simulink model "nonLin_Model_std_V2"  (R2023b)
settings: Solver=ode23t  StartTime=0.0  StopTime=Tend  FixedStep=Ts  MaxStep=0.002  RelTol=1e-3
InitFcn:
  | sysParam = load("sysParam.mat");
  | load('./zz_temp/controlletTypeToUse.mat')
undefined symbols (not defined in the file): C, sysID
libraries: slpidlib x12, cstblocks x2
(part 1 of 2)
settings Model: Creator=maxja  LastModifiedBy=maxja

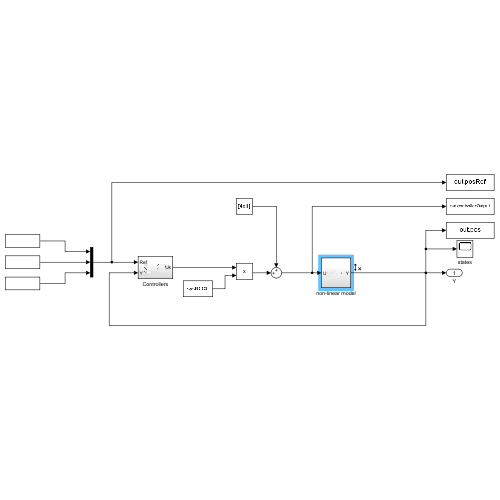
[thumbnail: Simulink's stored preview of the top-level diagram]
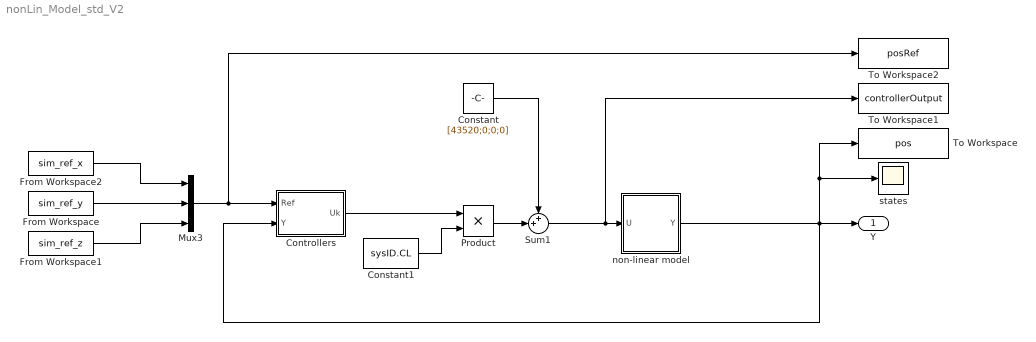
== system nonLin_Model_std_V2 ==
  Constant : Constant  Value=[43520;0;0;0]
  Constant1 : Constant  Value=sysID.CL
  Controllers : Subsystem
  From Workspace : FromWorkspace  VariableName=sim_ref_y
  From Workspace1 : FromWorkspace  VariableName=sim_ref_z
  From Workspace2 : FromWorkspace  VariableName=sim_ref_x
  Mux3 : Mux  Inputs=3
  Product : Product
  Sum1 : Sum  Inputs=++|
  To Workspace : ToWorkspace  VariableName=pos  SaveFormat=Timeseries  SampleTime=-1
  To Workspace1 : ToWorkspace  VariableName=controllerOutput  SaveFormat=Timeseries  SampleTime=-1
  To Workspace2 : ToWorkspace  VariableName=posRef  SaveFormat=Timeseries  SampleTime=-1
  non-linear model : Subsystem
  states : Scope
  Y : Outport
  wires:
  non-linear model/1(Y) -> To Workspace/1, states/1, Controllers/2(Y), Y/1
  From Workspace2/1 -> Mux3/1
  From Workspace/1 -> Mux3/2
  From Workspace1/1 -> Mux3/3
  Sum1/1 -> To Workspace1/1, non-linear model/1(U)
  Mux3/1 -> To Workspace2/1, Controllers/1(Ref)
  Controllers/1(Uk) -> Product/1
  Constant/1 -> Sum1/1
  Product/1 -> Sum1/2
  Constant1/1 -> Product/2

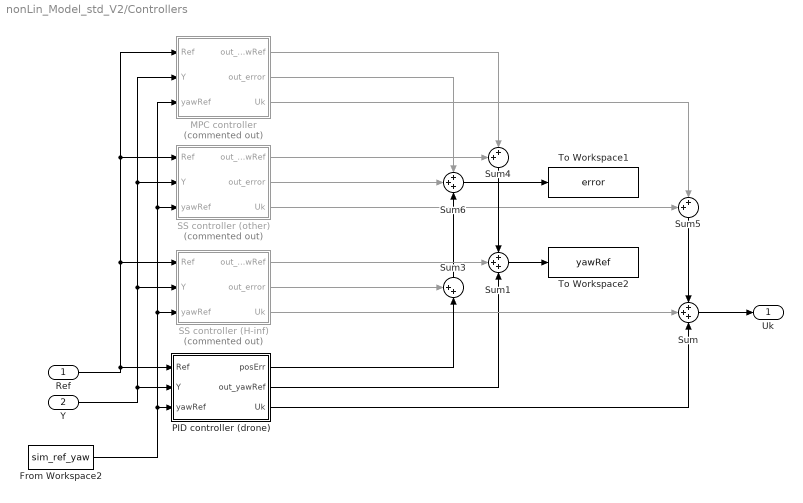
== system nonLin_Model_std_V2/Controllers ==
  Ref : Inport
  Y : Inport  Port=2
  From Workspace2 : FromWorkspace  VariableName=sim_ref_yaw
  MPC controller : Subsystem  Commented=on
  PID controller (drone) : Subsystem
  SS controller (H-inf) : Subsystem  Commented=on
  SS controller (other) : Subsystem  Commented=on
  Sum : Sum  Inputs=+++
  Sum1 : Sum  Inputs=+++
  Sum3 : Sum  Inputs=++|
  Sum4 : Sum  Inputs=++|
  Sum5 : Sum  Inputs=++|
  Sum6 : Sum  Inputs=+++
  To Workspace1 : ToWorkspace  VariableName=error  SaveFormat=Timeseries  SampleTime=-1
  To Workspace2 : ToWorkspace  VariableName=yawRef  SaveFormat=Timeseries  SampleTime=-1
  Uk : Outport
  wires:
  Y/1 -> PID controller (drone)/2(Y), SS controller (H-inf)/2(Y), MPC controller/2(Y), SS controller (other)/2(Y)
  Ref/1 -> PID controller (drone)/1(Ref), MPC controller/1(Ref), SS controller (other)/1(Ref), SS controller (H-inf)/1(Ref)
  SS controller (other)/3(Uk) -> Sum5/1
  PID controller (drone)/3(Uk) -> Sum/3
  From Workspace2/1 -> MPC controller/3(yawRef), SS controller (other)/3(yawRef), SS controller (H-inf)/3(yawRef), PID controller (drone)/3(yawRef)
  SS controller (other)/1(out_yawRef) -> Sum4/1
  SS controller (other)/2(out_error) -> Sum6/2
  Sum6/1 -> To Workspace1/1
  Sum1/1 -> To Workspace2/1
  PID controller (drone)/2(out_yawRef) -> Sum1/3
  SS controller (H-inf)/3(Uk) -> Sum/2
  Sum3/1 -> Sum6/3
  PID controller (drone)/1(posErr) -> Sum3/2
  MPC controller/1(out_yawRef) -> Sum4/2
  Sum4/1 -> Sum1/1
  Sum5/1 -> Sum/1
  MPC controller/3(Uk) -> Sum5/2
  MPC controller/2(out_error) -> Sum6/1
  SS controller (H-inf)/1(out_yawRef) -> Sum1/2
  SS controller (H-inf)/2(out_error) -> Sum3/1
  Sum/1 -> Uk/1

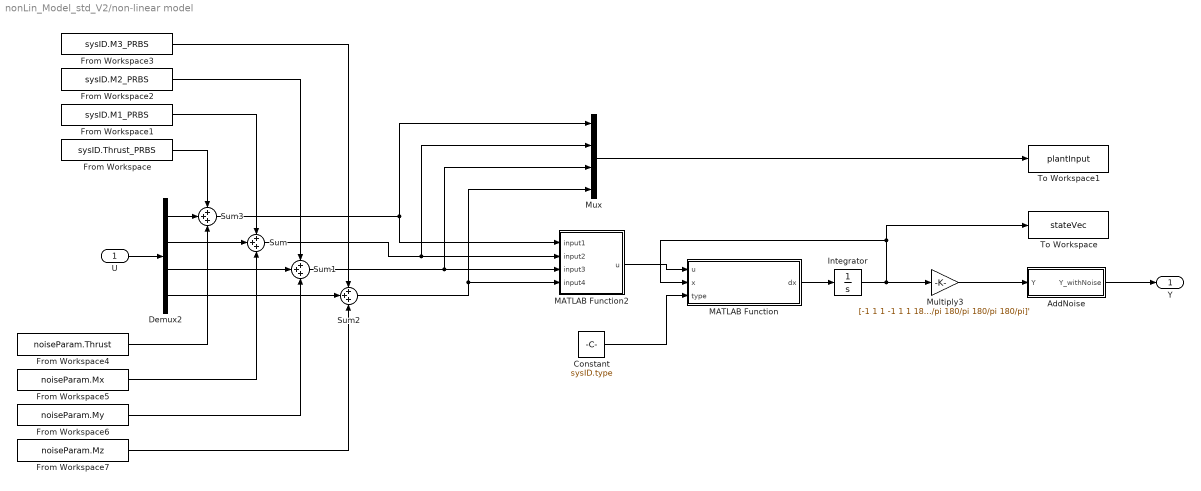
== system nonLin_Model_std_V2/non-linear model ==
  U : Inport  PortDimensions=4
  AddNoise : Subsystem
  Constant : Constant  Value=sysID.type
  Demux2 : Demux
  From Workspace : FromWorkspace  VariableName=sysID.Thrust_PRBS
  From Workspace1 : FromWorkspace  VariableName=sysID.M1_PRBS
  From Workspace2 : FromWorkspace  VariableName=sysID.M2_PRBS
  From Workspace3 : FromWorkspace  VariableName=sysID.M3_PRBS
  From Workspace4 : FromWorkspace  VariableName=noiseParam.Thrust
  From Workspace5 : FromWorkspace  VariableName=noiseParam.Mx
  From Workspace6 : FromWorkspace  VariableName=noiseParam.My
  From Workspace7 : FromWorkspace  VariableName=noiseParam.Mz
  Integrator : Integrator  InitialCondition=[0;0;0;0;0;0;0;0;0;0;0;0]  LimitOutput=on  UpperSaturationLimit=[inf inf inf inf inf inf inf inf inf inf inf inf]'  LowerSaturationLimit=-[inf inf 0 inf inf inf inf inf inf inf inf inf]'
  MATLAB Function : MATLAB Function  TreatAsAtomicUnit=on
  MATLAB Function2 : MATLAB Function  TreatAsAtomicUnit=on
  Multiply3 : Gain  Gain=[-1 1 1 -1 1 1 180/pi 180/pi 180/pi 180/pi 180/pi 180/pi]'
  Mux : Mux
  Sum{,1..3} (4 alike) : Sum  Inputs=+++
  To Workspace : ToWorkspace  VariableName=stateVec  SaveFormat=Timeseries  SampleTime=-1
  To Workspace1 : ToWorkspace  VariableName=plantInput  SaveFormat=Timeseries  SampleTime=-1
  Y : Outport
  wires:
  MATLAB Function/1(dx) -> Integrator/1
  U/1 -> Demux2/1
  Sum/1 -> Mux/2, MATLAB Function2/2(input2)
  Sum3/1 -> MATLAB Function2/1(input1), Mux/1
  Sum1/1 -> MATLAB Function2/3(input3), Mux/3
  Sum2/1 -> MATLAB Function2/4(input4), Mux/4
  From Workspace5/1 -> Sum/3
  From Workspace6/1 -> Sum1/3
  From Workspace7/1 -> Sum2/3
  From Workspace/1 -> Sum3/1
  From Workspace1/1 -> Sum/1
  From Workspace2/1 -> Sum1/1
  From Workspace3/1 -> Sum2/1
  Constant/1 -> MATLAB Function/3(type)
  Demux2/2 -> Sum/2
  Demux2/4 -> Sum2/2
  Demux2/3 -> Sum1/2
  Demux2/1 -> Sum3/2
  Multiply3/1 -> AddNoise/1(Y)
  MATLAB Function2/1(u) -> MATLAB Function/1(u)
  Mux/1 -> To Workspace1/1
  AddNoise/1(Y_withNoise) -> Y/1
  From Workspace4/1 -> Sum3/3
  Integrator/1 -> Multiply3/1, To Workspace/1, MATLAB Function/2(x)

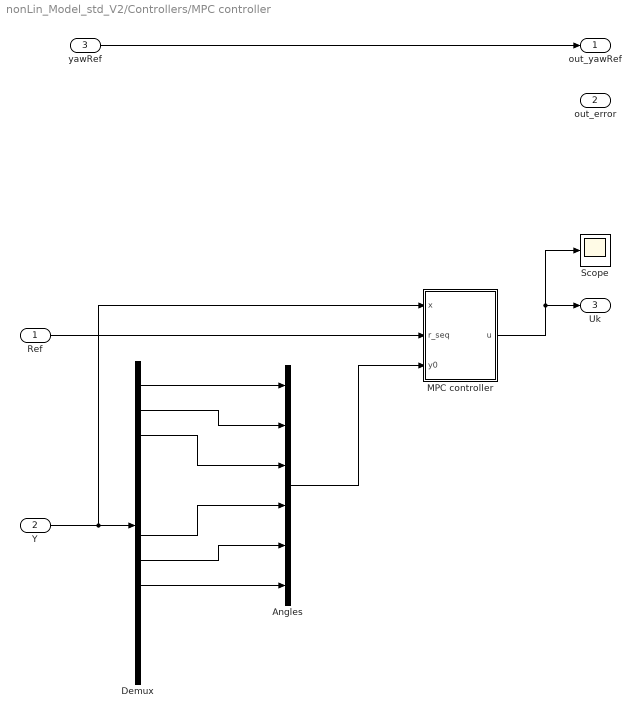
== system nonLin_Model_std_V2/Controllers/MPC controller ==
  Ref : Inport
  Y : Inport  Port=2
  yawRef : Inport  Port=3
  Angles : Mux  Inputs=6
  Demux : Demux  Outputs=12
  MPC controller : MATLAB Function  TreatAsAtomicUnit=on
  Scope : Scope
  out_yawRef : Outport
  out_error : Outport  Port=2
  Uk : Outport  Port=3
  wires:
  MPC controller/1(u) -> Scope/1, Uk/1
  Demux/7 -> Angles/4
  yawRef/1 -> out_yawRef/1
  Demux/9 -> Angles/6
  Demux/1 -> Angles/1
  Demux/3 -> Angles/3
  Demux/2 -> Angles/2
  Y/1 -> MPC controller/1(x), Demux/1
  Ref/1 -> MPC controller/2(r_seq)
  Demux/8 -> Angles/5
  Angles/1 -> MPC controller/3(y0)

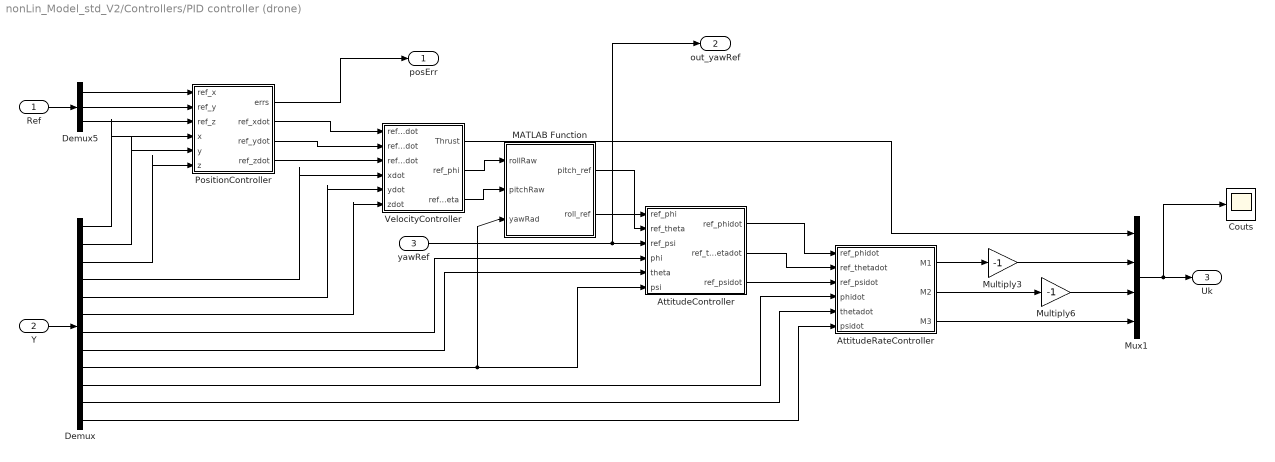
== system nonLin_Model_std_V2/Controllers/PID controller (drone) ==
  Ref : Inport
  Y : Inport  Port=2
  yawRef : Inport  Port=3
  AttitudeController : Subsystem
  AttitudeRateController : Subsystem
  Couts : Scope
  Demux : Demux  Outputs=12
  Demux5 : Demux  Outputs=3
  MATLAB Function : MATLAB Function  TreatAsAtomicUnit=on
  Multiply3 : Gain  Gain=-1
  Multiply6 : Gain  Gain=-1
  Mux1 : Mux
  PositionController : Subsystem
  VelocityController : Subsystem
  posErr : Outport
  out_yawRef : Outport  Port=2
  Uk : Outport  Port=3
  wires:
  Y/1 -> Demux/1
  Demux/1 -> PositionController/4(x)
  Demux/2 -> PositionController/5(y)
  Demux/3 -> PositionController/6(z)
  Demux/12 -> AttitudeRateController/6(psidot)
  Demux/11 -> AttitudeRateController/5(thetadot)
  Demux/10 -> AttitudeRateController/4(phidot)
  Demux/9 -> MATLAB Function/3(yawRad), AttitudeController/6(psi)
  Demux/6 -> VelocityController/6(zdot)
  Demux/5 -> VelocityController/5(ydot)
  Demux/4 -> VelocityController/4(xdot)
  Demux5/1 -> PositionController/1(ref_x)
  Demux5/2 -> PositionController/2(ref_y)
  Demux5/3 -> PositionController/3(ref_z)
  Ref/1 -> Demux5/1
  PositionController/2(ref_xdot) -> VelocityController/1(ref_xdot)
  PositionController/3(ref_ydot) -> VelocityController/2(ref_ydot)
  PositionController/4(ref_zdot) -> VelocityController/3(ref_zdot)
  yawRef/1 -> out_yawRef/1, AttitudeController/3(ref_psi)
  AttitudeController/3(ref_psidot) -> AttitudeRateController/3(ref_psidot)
  AttitudeController/2(ref_thetadot) -> AttitudeRateController/2(ref_thetadot)
  AttitudeController/1(ref_phidot) -> AttitudeRateController/1(ref_phidot)
  AttitudeRateController/1(M1) -> Multiply3/1
  AttitudeRateController/3(M3) -> Mux1/4
  VelocityController/1(Thrust) -> Mux1/1
  Mux1/1 -> Couts/1, Uk/1
  Multiply3/1 -> Mux1/2
  AttitudeRateController/2(M2) -> Multiply6/1
  Multiply6/1 -> Mux1/3
  Demux/7 -> AttitudeController/4(phi)
  Demux/8 -> AttitudeController/5(theta)
  VelocityController/2(ref_phi) -> MATLAB Function/1(rollRaw)
  VelocityController/3(ref_theta) -> MATLAB Function/2(pitchRaw)
  MATLAB Function/1(pitch_ref) -> AttitudeController/2(ref_theta)
  MATLAB Function/2(roll_ref) -> AttitudeController/1(ref_phi)
  PositionController/1(errs) -> posErr/1

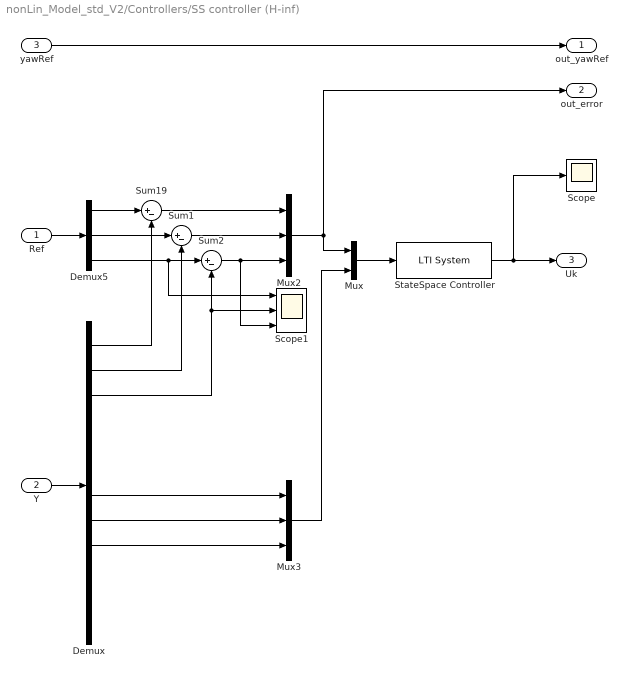
== system nonLin_Model_std_V2/Controllers/SS controller (H-inf) ==
  Ref : Inport
  Y : Inport  Port=2
  yawRef : Inport  Port=3
  Demux : Demux  Outputs=12
  Demux5 : Demux  Outputs=3
  Mux : Mux  Inputs=2
  Mux2 : Mux  Inputs=3
  Mux3 : Mux  Inputs=3
  Scope : Scope
  Scope1 : Scope  NumInputPorts=3
  StateSpace Controller : cstblocks/LTI System  sys=K  IC=[]  PadeOrder=0
  Sum1 : Sum  Inputs=|+-
  Sum19 : Sum  Inputs=|+-
  Sum2 : Sum  Inputs=|+-
  out_yawRef : Outport
  out_error : Outport  Port=2
  Uk : Outport  Port=3
  wires:
  Y/1 -> Demux/1
  Ref/1 -> Demux5/1
  Demux5/1 -> Sum19/1
  Demux5/2 -> Sum1/1
  Demux/3 -> Sum2/2, Scope1/2
  Demux/2 -> Sum1/2
  Sum19/1 -> Mux2/1
  Demux/1 -> Sum19/2
  Demux5/3 -> Scope1/1, Sum2/1
  Sum1/1 -> Mux2/2
  Sum2/1 -> Scope1/3, Mux2/3
  yawRef/1 -> out_yawRef/1
  Demux/9 -> Mux3/3
  Mux2/1 -> out_error/1, Mux/1
  Demux/7 -> Mux3/1
  Demux/8 -> Mux3/2
  Mux3/1 -> Mux/2
  Mux/1 -> StateSpace Controller/1
  StateSpace Controller/1 -> Uk/1, Scope/1

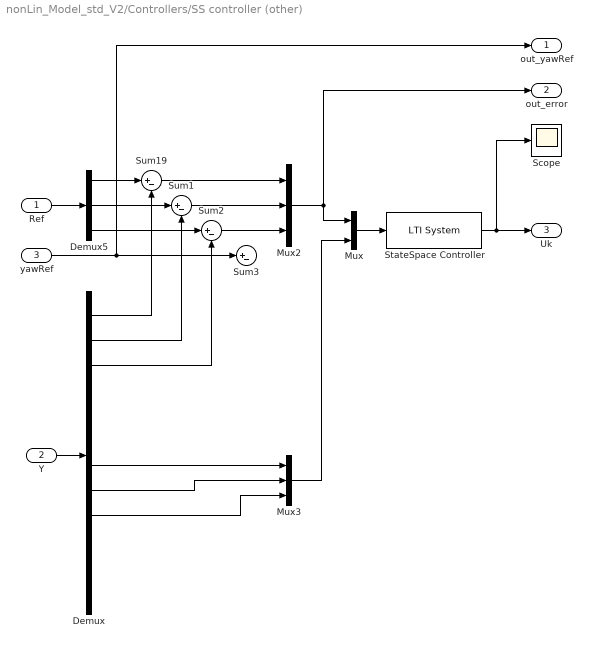
== system nonLin_Model_std_V2/Controllers/SS controller (other) ==
  Ref : Inport
  Y : Inport  Port=2
  yawRef : Inport  Port=3
  Demux : Demux  Outputs=12
  Demux5 : Demux  Outputs=3
  Mux : Mux  Inputs=2
  Mux2 : Mux  Inputs=3
  Mux3 : Mux  Inputs=3
  Scope : Scope
  StateSpace Controller : cstblocks/LTI System  sys=K  IC=[]  PadeOrder=0
  Sum{1..3,19} (4 alike) : Sum  Inputs=|+-
  out_yawRef : Outport
  out_error : Outport  Port=2
  Uk : Outport  Port=3
  wires:
  Y/1 -> Demux/1
  Ref/1 -> Demux5/1
  Demux5/1 -> Sum19/1
  Demux5/2 -> Sum1/1
  Demux/3 -> Sum2/2
  Demux/2 -> Sum1/2
  Sum19/1 -> Mux2/1
  Demux/1 -> Sum19/2
  Demux5/3 -> Sum2/1
  Sum1/1 -> Mux2/2
  Sum2/1 -> Mux2/3
  yawRef/1 -> out_yawRef/1, Sum3/1
  Demux/9 -> Mux3/3
  Mux2/1 -> Mux/1, out_error/1
  Demux/7 -> Mux3/1
  Demux/8 -> Mux3/2
  Mux3/1 -> Mux/2
  Mux/1 -> StateSpace Controller/1
  StateSpace Controller/1 -> Scope/1, Uk/1

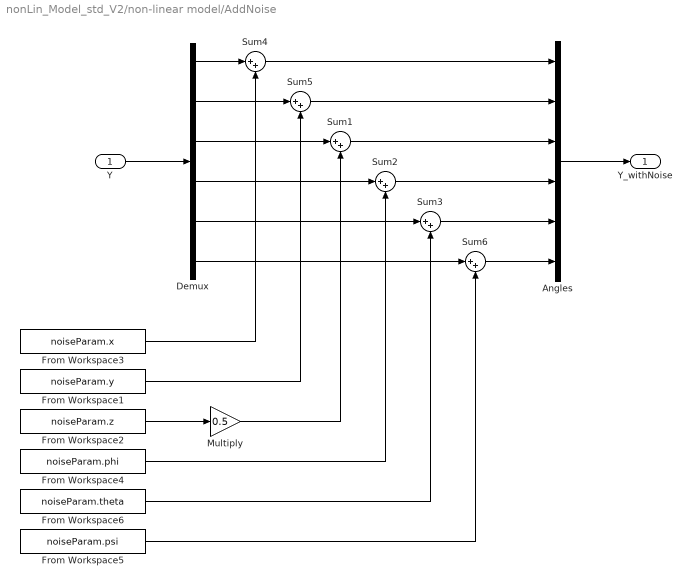
== system nonLin_Model_std_V2/non-linear model/AddNoise ==
  Y : Inport
  Angles : Mux  Inputs=6
  Demux : Demux  Outputs=6
  From Workspace1 : FromWorkspace  VariableName=noiseParam.y
  From Workspace2 : FromWorkspace  VariableName=noiseParam.z
  From Workspace3 : FromWorkspace  VariableName=noiseParam.x
  From Workspace4 : FromWorkspace  VariableName=noiseParam.phi
  From Workspace5 : FromWorkspace  VariableName=noiseParam.psi
  From Workspace6 : FromWorkspace  VariableName=noiseParam.theta
  Multiply : Gain  Gain=0.5
  Sum{1..6} (6 alike) : Sum  Inputs=|++
  Y_withNoise : Outport
  wires:
  Demux/2 -> Sum5/1
  Demux/6 -> Sum6/1
  Demux/1 -> Sum4/1
  Demux/3 -> Sum1/1
  Demux/4 -> Sum2/1
  Demux/5 -> Sum3/1
  Sum4/1 -> Angles/1
  Sum6/1 -> Angles/6
  Sum3/1 -> Angles/5
  Sum2/1 -> Angles/4
  Sum1/1 -> Angles/3
  Sum5/1 -> Angles/2
  Y/1 -> Demux/1
  Angles/1 -> Y_withNoise/1
  From Workspace3/1 -> Sum4/2
  From Workspace1/1 -> Sum5/2
  From Workspace2/1 -> Multiply/1
  From Workspace4/1 -> Sum2/2
  From Workspace6/1 -> Sum3/2
  From Workspace5/1 -> Sum6/2
  Multiply/1 -> Sum1/2

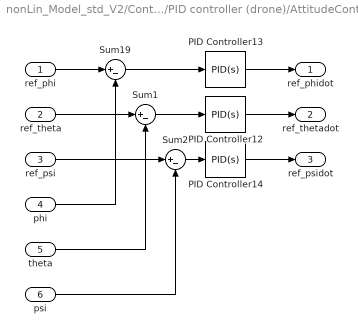
== system nonLin_Model_std_V2/Controllers/PID controller (drone)/AttitudeController ==
  ref_phi : Inport
  ref_theta : Inport  Port=2
  ref_psi : Inport  Port=3
  phi : Inport  Port=4
  theta : Inport  Port=5
  psi : Inport  Port=6
  PID Controller12 : slpidlib/PID Controller  Controller=PID  Form=Parallel  TimeDomain=Continuous-time  UseExternalTs=off  SampleTime=-1  IntegratorMethod=Forward Euler  FilterMethod=Forward Euler  ControllerParametersSource=internal  P=C.att.theta.Kp  I=C.att.theta.Ki  UseKiTs=off  D=C.att.theta.Kd  N=100  UseFilter=on  TunerSelectOption=Transfer Function Based (PID Tuner App)  InitialConditionSource=internal  InitialConditionForIntegrator=0  InitialConditionForFilter=0  DifferentiatorICPrevScaledInput=0  ExternalReset=none  TrackingMode=off  Kt=1  LimitOutput=off  SatLimitsSource=internal  UpperSaturationLimit=inf  LowerSaturationLimit=-inf  LinearizeAsGain=on  AntiWindupMode=none  Kb=1  LimitIntegrator=off  UpperIntegratorSaturationLimit=inf  LowerIntegratorSaturationLimit=-inf  POutMin=[]  POutMax=[]  IOutMin=[]  IOutMax=[]  DOutMin=[]  DOutMax=[]  NOutMin=[]  NOutMax=[]  SumOutMin=[]  SumOutMax=[]  SaturationOutMin=[]  SaturationOutMax=[]  PParamMin=[]  PParamMax=[]  IParamMin=[]  IParamMax=[]  DParamMin=[]  DParamMax=[]  NParamMin=[]  NParamMax=[]  KbParamMin=[]  KbParamMax=[]  KtParamMin=[]  KtParamMax=[]  KbOutMin=[]  KbOutMax=[]  KtOutMin=[]  KtOutMax=[]  IntegratorOutMin=[]  IntegratorOutMax=[]  FilterOutMin=[]  FilterOutMax=[]  SumI1OutMin=[]  SumI1OutMax=[]  SumI2OutMin=[]  SumI2OutMax=[]  SumI3OutMin=[]  SumI3OutMax=[]  SumI4OutMin=[]  SumI4OutMax=[]  SumDOutMin=[]  SumDOutMax=[]  DifferentiatorOutMin=[]  DifferentiatorOutMax=[]  FilterDiffOutCoefMin=[]  FilterDiffOutCoefMax=[]  ReciprocalOutMin=[]  ReciprocalOutMax=[]  SumDenOutMin=[]  SumDenOutMax=[]  SumNumOutMin=[]  SumNumOutMax=[]  DivideOutMin=[]  DivideOutMax=[]  UdiffTsProdOutMin=[]  UdiffTsProdOutMax=[]  NTsProdOutMin=[]  NTsProdOutMax=[]  UintegralTsProdOutMin=[]  UintegralTsProdOutMax=[]  UngainTsProdOutMin=[]  UngainTsProdOutMax=[]  ClampingZeroOutDataTypeStr=Inherit: Inherit via back propagation  ClampingZeroOutMin=[]  ClampingZeroOutMax=[]  FilterDenConstantOutDataTypeStr=Inherit: Inherit via back propagation  FilterDenConstantOutMin=[]  FilterDenConstantOutMax=[]  PCopyOutDataTypeStr=Inherit: Inherit via back propagation  PCopyOutMin=[]  PCopyOutMax=[]  NCopyOutDataTypeStr=Inherit: Inherit via back propagation  NCopyOutMin=[]  NCopyOutMax=[]  IntegratorContinuousStateAttributes=''  IntegratorStateMustResolveToSignalObject=off  IntegratorRTWStateStorageClass=Auto  FilterContinuousStateAttributes=''  FilterStateMustResolveToSignalObject=off  FilterRTWStateStorageClass=Auto  ParallelPVariant=InternalParameters  IdealPVariant=Disabled  IVariant=InternalParameters  DVariant=InternalParameters  IntegratorVariant=Continuous  SatVariant=Disabled  AWVariant=Passthrough  PCopyVariant=Disabled  TRVariant=Disabled  FdbkBlocksVariant=Forward  IdealPFdbkVariant=Disabled  SatFdbkVariant=Disabled  DerivativeFilterVariant=ContFilter  NVariant=InternalParameters  NCopyVariant=Disabled  FilterICVariant=InternalICsFilter  IntegratorICVariant=InternalICs  ExternalResetVariant=Disabled  TRSumVariant=Passthrough  SumFdbkVariant=Disabled  SumVariant=Sum_PID  TsampFilterVariant=InternalTs  TsampNgainVariant=Passthrough  TsampIntegralVariant=Disabled_SignalSpec  ExternalSaturationOutDataTypeStr=Inherit: Same as second input
  PID Controller13 : slpidlib/PID Controller  Controller=PID  Form=Parallel  TimeDomain=Continuous-time  UseExternalTs=off  SampleTime=-1  IntegratorMethod=Forward Euler  FilterMethod=Forward Euler  ControllerParametersSource=internal  P=C.att.phi.Kp  I=C.att.phi.Ki  UseKiTs=off  D=C.att.phi.Kd  N=100  UseFilter=on  TunerSelectOption=Transfer Function Based (PID Tuner App)  InitialConditionSource=internal  InitialConditionForIntegrator=0  InitialConditionForFilter=0  DifferentiatorICPrevScaledInput=0  ExternalReset=none  TrackingMode=off  Kt=1  LimitOutput=off  SatLimitsSource=internal  UpperSaturationLimit=inf  LowerSaturationLimit=-inf  LinearizeAsGain=on  AntiWindupMode=none  Kb=1  LimitIntegrator=off  UpperIntegratorSaturationLimit=inf  LowerIntegratorSaturationLimit=-inf  POutMin=[]  POutMax=[]  IOutMin=[]  IOutMax=[]  DOutMin=[]  DOutMax=[]  NOutMin=[]  NOutMax=[]  SumOutMin=[]  SumOutMax=[]  SaturationOutMin=[]  SaturationOutMax=[]  PParamMin=[]  PParamMax=[]  IParamMin=[]  IParamMax=[]  DParamMin=[]  DParamMax=[]  NParamMin=[]  NParamMax=[]  KbParamMin=[]  KbParamMax=[]  KtParamMin=[]  KtParamMax=[]  KbOutMin=[]  KbOutMax=[]  KtOutMin=[]  KtOutMax=[]  IntegratorOutMin=[]  IntegratorOutMax=[]  FilterOutMin=[]  FilterOutMax=[]  SumI1OutMin=[]  SumI1OutMax=[]  SumI2OutMin=[]  SumI2OutMax=[]  SumI3OutMin=[]  SumI3OutMax=[]  SumI4OutMin=[]  SumI4OutMax=[]  SumDOutMin=[]  SumDOutMax=[]  DifferentiatorOutMin=[]  DifferentiatorOutMax=[]  FilterDiffOutCoefMin=[]  FilterDiffOutCoefMax=[]  ReciprocalOutMin=[]  ReciprocalOutMax=[]  SumDenOutMin=[]  SumDenOutMax=[]  SumNumOutMin=[]  SumNumOutMax=[]  DivideOutMin=[]  DivideOutMax=[]  UdiffTsProdOutMin=[]  UdiffTsProdOutMax=[]  NTsProdOutMin=[]  NTsProdOutMax=[]  UintegralTsProdOutMin=[]  UintegralTsProdOutMax=[]  UngainTsProdOutMin=[]  UngainTsProdOutMax=[]  ClampingZeroOutDataTypeStr=Inherit: Inherit via back propagation  ClampingZeroOutMin=[]  ClampingZeroOutMax=[]  FilterDenConstantOutDataTypeStr=Inherit: Inherit via back propagation  FilterDenConstantOutMin=[]  FilterDenConstantOutMax=[]  PCopyOutDataTypeStr=Inherit: Inherit via back propagation  PCopyOutMin=[]  PCopyOutMax=[]  NCopyOutDataTypeStr=Inherit: Inherit via back propagation  NCopyOutMin=[]  NCopyOutMax=[]  IntegratorContinuousStateAttributes=''  IntegratorStateMustResolveToSignalObject=off  IntegratorRTWStateStorageClass=Auto  FilterContinuousStateAttributes=''  FilterStateMustResolveToSignalObject=off  FilterRTWStateStorageClass=Auto  ParallelPVariant=InternalParameters  IdealPVariant=Disabled  IVariant=InternalParameters  DVariant=InternalParameters  IntegratorVariant=Continuous  SatVariant=Disabled  AWVariant=Passthrough  PCopyVariant=Disabled  TRVariant=Disabled  FdbkBlocksVariant=Forward  IdealPFdbkVariant=Disabled  SatFdbkVariant=Disabled  DerivativeFilterVariant=ContFilter  NVariant=InternalParameters  NCopyVariant=Disabled  FilterICVariant=InternalICsFilter  IntegratorICVariant=InternalICs  ExternalResetVariant=Disabled  TRSumVariant=Passthrough  SumFdbkVariant=Disabled  SumVariant=Sum_PID  TsampFilterVariant=InternalTs  TsampNgainVariant=Passthrough  TsampIntegralVariant=Disabled_SignalSpec  ExternalSaturationOutDataTypeStr=Inherit: Same as second input
  PID Controller14 : slpidlib/PID Controller  Controller=PID  Form=Parallel  TimeDomain=Continuous-time  UseExternalTs=off  SampleTime=-1  IntegratorMethod=Forward Euler  FilterMethod=Forward Euler  ControllerParametersSource=internal  P=C.att.psi.Kp  I=C.att.psi.Ki  UseKiTs=off  D=C.att.psi.Kd  N=100  UseFilter=on  TunerSelectOption=Transfer Function Based (PID Tuner App)  InitialConditionSource=internal  InitialConditionForIntegrator=0  InitialConditionForFilter=0  DifferentiatorICPrevScaledInput=0  ExternalReset=none  TrackingMode=off  Kt=1  LimitOutput=off  SatLimitsSource=internal  UpperSaturationLimit=inf  LowerSaturationLimit=-inf  LinearizeAsGain=on  AntiWindupMode=none  Kb=1  LimitIntegrator=off  UpperIntegratorSaturationLimit=inf  LowerIntegratorSaturationLimit=-inf  POutMin=[]  POutMax=[]  IOutMin=[]  IOutMax=[]  DOutMin=[]  DOutMax=[]  NOutMin=[]  NOutMax=[]  SumOutMin=[]  SumOutMax=[]  SaturationOutMin=[]  SaturationOutMax=[]  PParamMin=[]  PParamMax=[]  IParamMin=[]  IParamMax=[]  DParamMin=[]  DParamMax=[]  NParamMin=[]  NParamMax=[]  KbParamMin=[]  KbParamMax=[]  KtParamMin=[]  KtParamMax=[]  KbOutMin=[]  KbOutMax=[]  KtOutMin=[]  KtOutMax=[]  IntegratorOutMin=[]  IntegratorOutMax=[]  FilterOutMin=[]  FilterOutMax=[]  SumI1OutMin=[]  SumI1OutMax=[]  SumI2OutMin=[]  SumI2OutMax=[]  SumI3OutMin=[]  SumI3OutMax=[]  SumI4OutMin=[]  SumI4OutMax=[]  SumDOutMin=[]  SumDOutMax=[]  DifferentiatorOutMin=[]  DifferentiatorOutMax=[]  FilterDiffOutCoefMin=[]  FilterDiffOutCoefMax=[]  ReciprocalOutMin=[]  ReciprocalOutMax=[]  SumDenOutMin=[]  SumDenOutMax=[]  SumNumOutMin=[]  SumNumOutMax=[]  DivideOutMin=[]  DivideOutMax=[]  UdiffTsProdOutMin=[]  UdiffTsProdOutMax=[]  NTsProdOutMin=[]  NTsProdOutMax=[]  UintegralTsProdOutMin=[]  UintegralTsProdOutMax=[]  UngainTsProdOutMin=[]  UngainTsProdOutMax=[]  ClampingZeroOutDataTypeStr=Inherit: Inherit via back propagation  ClampingZeroOutMin=[]  ClampingZeroOutMax=[]  FilterDenConstantOutDataTypeStr=Inherit: Inherit via back propagation  FilterDenConstantOutMin=[]  FilterDenConstantOutMax=[]  PCopyOutDataTypeStr=Inherit: Inherit via back propagation  PCopyOutMin=[]  PCopyOutMax=[]  NCopyOutDataTypeStr=Inherit: Inherit via back propagation  NCopyOutMin=[]  NCopyOutMax=[]  IntegratorContinuousStateAttributes=''  IntegratorStateMustResolveToSignalObject=off  IntegratorRTWStateStorageClass=Auto  FilterContinuousStateAttributes=''  FilterStateMustResolveToSignalObject=off  FilterRTWStateStorageClass=Auto  ParallelPVariant=InternalParameters  IdealPVariant=Disabled  IVariant=InternalParameters  DVariant=InternalParameters  IntegratorVariant=Continuous  SatVariant=Disabled  AWVariant=Passthrough  PCopyVariant=Disabled  TRVariant=Disabled  FdbkBlocksVariant=Forward  IdealPFdbkVariant=Disabled  SatFdbkVariant=Disabled  DerivativeFilterVariant=ContFilter  NVariant=InternalParameters  NCopyVariant=Disabled  FilterICVariant=InternalICsFilter  IntegratorICVariant=InternalICs  ExternalResetVariant=Disabled  TRSumVariant=Passthrough  SumFdbkVariant=Disabled  SumVariant=Sum_PID  TsampFilterVariant=InternalTs  TsampNgainVariant=Passthrough  TsampIntegralVariant=Disabled_SignalSpec  ExternalSaturationOutDataTypeStr=Inherit: Same as second input
  Sum1 : Sum  Inputs=|+-
  Sum19 : Sum  Inputs=|+-
  Sum2 : Sum  Inputs=|+-
  ref_phidot : Outport
  ref_thetadot : Outport  Port=2
  ref_psidot : Outport  Port=3
  wires:
  phi/1 -> Sum19/2
  Sum19/1 -> PID Controller13/1
  Sum1/1 -> PID Controller12/1
  PID Controller12/1 -> ref_thetadot/1
  psi/1 -> Sum2/2
  Sum2/1 -> PID Controller14/1
  theta/1 -> Sum1/2
  PID Controller13/1 -> ref_phidot/1
  ref_phi/1 -> Sum19/1
  ref_theta/1 -> Sum1/1
  ref_psi/1 -> Sum2/1
  PID Controller14/1 -> ref_psidot/1

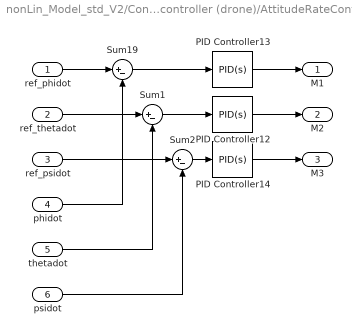
== system nonLin_Model_std_V2/Controllers/PID controller (drone)/AttitudeRateController ==
  ref_phidot : Inport
  ref_thetadot : Inport  Port=2
  ref_psidot : Inport  Port=3
  phidot : Inport  Port=4
  thetadot : Inport  Port=5
  psidot : Inport  Port=6
  PID Controller12 : slpidlib/PID Controller  Controller=PID  Form=Parallel  TimeDomain=Continuous-time  UseExternalTs=off  SampleTime=-1  IntegratorMethod=Forward Euler  FilterMethod=Forward Euler  ControllerParametersSource=internal  P=C.attRate.thetadot.Kp  I=C.attRate.thetadot.Ki  UseKiTs=off  D=C.attRate.thetadot.Kd  N=100  UseFilter=on  TunerSelectOption=Transfer Function Based (PID Tuner App)  InitialConditionSource=internal  InitialConditionForIntegrator=0  InitialConditionForFilter=0  DifferentiatorICPrevScaledInput=0  ExternalReset=none  TrackingMode=off  Kt=1  LimitOutput=off  SatLimitsSource=internal  UpperSaturationLimit=inf  LowerSaturationLimit=-inf  LinearizeAsGain=on  AntiWindupMode=none  Kb=1  LimitIntegrator=off  UpperIntegratorSaturationLimit=inf  LowerIntegratorSaturationLimit=-inf  POutMin=[]  POutMax=[]  IOutMin=[]  IOutMax=[]  DOutMin=[]  DOutMax=[]  NOutMin=[]  NOutMax=[]  SumOutMin=[]  SumOutMax=[]  SaturationOutMin=[]  SaturationOutMax=[]  PParamMin=[]  PParamMax=[]  IParamMin=[]  IParamMax=[]  DParamMin=[]  DParamMax=[]  NParamMin=[]  NParamMax=[]  KbParamMin=[]  KbParamMax=[]  KtParamMin=[]  KtParamMax=[]  KbOutMin=[]  KbOutMax=[]  KtOutMin=[]  KtOutMax=[]  IntegratorOutMin=[]  IntegratorOutMax=[]  FilterOutMin=[]  FilterOutMax=[]  SumI1OutMin=[]  SumI1OutMax=[]  SumI2OutMin=[]  SumI2OutMax=[]  SumI3OutMin=[]  SumI3OutMax=[]  SumI4OutMin=[]  SumI4OutMax=[]  SumDOutMin=[]  SumDOutMax=[]  DifferentiatorOutMin=[]  DifferentiatorOutMax=[]  FilterDiffOutCoefMin=[]  FilterDiffOutCoefMax=[]  ReciprocalOutMin=[]  ReciprocalOutMax=[]  SumDenOutMin=[]  SumDenOutMax=[]  SumNumOutMin=[]  SumNumOutMax=[]  DivideOutMin=[]  DivideOutMax=[]  UdiffTsProdOutMin=[]  UdiffTsProdOutMax=[]  NTsProdOutMin=[]  NTsProdOutMax=[]  UintegralTsProdOutMin=[]  UintegralTsProdOutMax=[]  UngainTsProdOutMin=[]  UngainTsProdOutMax=[]  ClampingZeroOutDataTypeStr=Inherit: Inherit via back propagation  ClampingZeroOutMin=[]  ClampingZeroOutMax=[]  FilterDenConstantOutDataTypeStr=Inherit: Inherit via back propagation  FilterDenConstantOutMin=[]  FilterDenConstantOutMax=[]  PCopyOutDataTypeStr=Inherit: Inherit via back propagation  PCopyOutMin=[]  PCopyOutMax=[]  NCopyOutDataTypeStr=Inherit: Inherit via back propagation  NCopyOutMin=[]  NCopyOutMax=[]  IntegratorContinuousStateAttributes=''  IntegratorStateMustResolveToSignalObject=off  IntegratorRTWStateStorageClass=Auto  FilterContinuousStateAttributes=''  FilterStateMustResolveToSignalObject=off  FilterRTWStateStorageClass=Auto  ParallelPVariant=InternalParameters  IdealPVariant=Disabled  IVariant=InternalParameters  DVariant=InternalParameters  IntegratorVariant=Continuous  SatVariant=Disabled  AWVariant=Passthrough  PCopyVariant=Disabled  TRVariant=Disabled  FdbkBlocksVariant=Forward  IdealPFdbkVariant=Disabled  SatFdbkVariant=Disabled  DerivativeFilterVariant=ContFilter  NVariant=InternalParameters  NCopyVariant=Disabled  FilterICVariant=InternalICsFilter  IntegratorICVariant=InternalICs  ExternalResetVariant=Disabled  TRSumVariant=Passthrough  SumFdbkVariant=Disabled  SumVariant=Sum_PID  TsampFilterVariant=InternalTs  TsampNgainVariant=Passthrough  TsampIntegralVariant=Disabled_SignalSpec  ExternalSaturationOutDataTypeStr=Inherit: Same as second input
  PID Controller13 : slpidlib/PID Controller  Controller=PID  Form=Parallel  TimeDomain=Continuous-time  UseExternalTs=off  SampleTime=-1  IntegratorMethod=Forward Euler  FilterMethod=Forward Euler  ControllerParametersSource=internal  P=C.attRate.phidot.Kp  I=C.attRate.phidot.Ki  UseKiTs=off  D=C.attRate.phidot.Kd  N=100  UseFilter=on  TunerSelectOption=Transfer Function Based (PID Tuner App)  InitialConditionSource=internal  InitialConditionForIntegrator=0  InitialConditionForFilter=0  DifferentiatorICPrevScaledInput=0  ExternalReset=none  TrackingMode=off  Kt=1  LimitOutput=off  SatLimitsSource=internal  UpperSaturationLimit=inf  LowerSaturationLimit=-inf  LinearizeAsGain=on  AntiWindupMode=none  Kb=1  LimitIntegrator=off  UpperIntegratorSaturationLimit=inf  LowerIntegratorSaturationLimit=-inf  POutMin=[]  POutMax=[]  IOutMin=[]  IOutMax=[]  DOutMin=[]  DOutMax=[]  NOutMin=[]  NOutMax=[]  SumOutMin=[]  SumOutMax=[]  SaturationOutMin=[]  SaturationOutMax=[]  PParamMin=[]  PParamMax=[]  IParamMin=[]  IParamMax=[]  DParamMin=[]  DParamMax=[]  NParamMin=[]  NParamMax=[]  KbParamMin=[]  KbParamMax=[]  KtParamMin=[]  KtParamMax=[]  KbOutMin=[]  KbOutMax=[]  KtOutMin=[]  KtOutMax=[]  IntegratorOutMin=[]  IntegratorOutMax=[]  FilterOutMin=[]  FilterOutMax=[]  SumI1OutMin=[]  SumI1OutMax=[]  SumI2OutMin=[]  SumI2OutMax=[]  SumI3OutMin=[]  SumI3OutMax=[]  SumI4OutMin=[]  SumI4OutMax=[]  SumDOutMin=[]  SumDOutMax=[]  DifferentiatorOutMin=[]  DifferentiatorOutMax=[]  FilterDiffOutCoefMin=[]  FilterDiffOutCoefMax=[]  ReciprocalOutMin=[]  ReciprocalOutMax=[]  SumDenOutMin=[]  SumDenOutMax=[]  SumNumOutMin=[]  SumNumOutMax=[]  DivideOutMin=[]  DivideOutMax=[]  UdiffTsProdOutMin=[]  UdiffTsProdOutMax=[]  NTsProdOutMin=[]  NTsProdOutMax=[]  UintegralTsProdOutMin=[]  UintegralTsProdOutMax=[]  UngainTsProdOutMin=[]  UngainTsProdOutMax=[]  ClampingZeroOutDataTypeStr=Inherit: Inherit via back propagation  ClampingZeroOutMin=[]  ClampingZeroOutMax=[]  FilterDenConstantOutDataTypeStr=Inherit: Inherit via back propagation  FilterDenConstantOutMin=[]  FilterDenConstantOutMax=[]  PCopyOutDataTypeStr=Inherit: Inherit via back propagation  PCopyOutMin=[]  PCopyOutMax=[]  NCopyOutDataTypeStr=Inherit: Inherit via back propagation  NCopyOutMin=[]  NCopyOutMax=[]  IntegratorContinuousStateAttributes=''  IntegratorStateMustResolveToSignalObject=off  IntegratorRTWStateStorageClass=Auto  FilterContinuousStateAttributes=''  FilterStateMustResolveToSignalObject=off  FilterRTWStateStorageClass=Auto  ParallelPVariant=InternalParameters  IdealPVariant=Disabled  IVariant=InternalParameters  DVariant=InternalParameters  IntegratorVariant=Continuous  SatVariant=Disabled  AWVariant=Passthrough  PCopyVariant=Disabled  TRVariant=Disabled  FdbkBlocksVariant=Forward  IdealPFdbkVariant=Disabled  SatFdbkVariant=Disabled  DerivativeFilterVariant=ContFilter  NVariant=InternalParameters  NCopyVariant=Disabled  FilterICVariant=InternalICsFilter  IntegratorICVariant=InternalICs  ExternalResetVariant=Disabled  TRSumVariant=Passthrough  SumFdbkVariant=Disabled  SumVariant=Sum_PID  TsampFilterVariant=InternalTs  TsampNgainVariant=Passthrough  TsampIntegralVariant=Disabled_SignalSpec  ExternalSaturationOutDataTypeStr=Inherit: Same as second input
  PID Controller14 : slpidlib/PID Controller  Controller=PID  Form=Parallel  TimeDomain=Continuous-time  UseExternalTs=off  SampleTime=-1  IntegratorMethod=Forward Euler  FilterMethod=Forward Euler  ControllerParametersSource=internal  P=C.attRate.psidot.Kp  I=C.attRate.psidot.Ki  UseKiTs=off  D=C.attRate.psidot.Kd  N=100  UseFilter=on  TunerSelectOption=Transfer Function Based (PID Tuner App)  InitialConditionSource=internal  InitialConditionForIntegrator=0  InitialConditionForFilter=0  DifferentiatorICPrevScaledInput=0  ExternalReset=none  TrackingMode=off  Kt=1  LimitOutput=off  SatLimitsSource=internal  UpperSaturationLimit=inf  LowerSaturationLimit=-inf  LinearizeAsGain=on  AntiWindupMode=none  Kb=1  LimitIntegrator=off  UpperIntegratorSaturationLimit=inf  LowerIntegratorSaturationLimit=-inf  POutMin=[]  POutMax=[]  IOutMin=[]  IOutMax=[]  DOutMin=[]  DOutMax=[]  NOutMin=[]  NOutMax=[]  SumOutMin=[]  SumOutMax=[]  SaturationOutMin=[]  SaturationOutMax=[]  PParamMin=[]  PParamMax=[]  IParamMin=[]  IParamMax=[]  DParamMin=[]  DParamMax=[]  NParamMin=[]  NParamMax=[]  KbParamMin=[]  KbParamMax=[]  KtParamMin=[]  KtParamMax=[]  KbOutMin=[]  KbOutMax=[]  KtOutMin=[]  KtOutMax=[]  IntegratorOutMin=[]  IntegratorOutMax=[]  FilterOutMin=[]  FilterOutMax=[]  SumI1OutMin=[]  SumI1OutMax=[]  SumI2OutMin=[]  SumI2OutMax=[]  SumI3OutMin=[]  SumI3OutMax=[]  SumI4OutMin=[]  SumI4OutMax=[]  SumDOutMin=[]  SumDOutMax=[]  DifferentiatorOutMin=[]  DifferentiatorOutMax=[]  FilterDiffOutCoefMin=[]  FilterDiffOutCoefMax=[]  ReciprocalOutMin=[]  ReciprocalOutMax=[]  SumDenOutMin=[]  SumDenOutMax=[]  SumNumOutMin=[]  SumNumOutMax=[]  DivideOutMin=[]  DivideOutMax=[]  UdiffTsProdOutMin=[]  UdiffTsProdOutMax=[]  NTsProdOutMin=[]  NTsProdOutMax=[]  UintegralTsProdOutMin=[]  UintegralTsProdOutMax=[]  UngainTsProdOutMin=[]  UngainTsProdOutMax=[]  ClampingZeroOutDataTypeStr=Inherit: Inherit via back propagation  ClampingZeroOutMin=[]  ClampingZeroOutMax=[]  FilterDenConstantOutDataTypeStr=Inherit: Inherit via back propagation  FilterDenConstantOutMin=[]  FilterDenConstantOutMax=[]  PCopyOutDataTypeStr=Inherit: Inherit via back propagation  PCopyOutMin=[]  PCopyOutMax=[]  NCopyOutDataTypeStr=Inherit: Inherit via back propagation  NCopyOutMin=[]  NCopyOutMax=[]  IntegratorContinuousStateAttributes=''  IntegratorStateMustResolveToSignalObject=off  IntegratorRTWStateStorageClass=Auto  FilterContinuousStateAttributes=''  FilterStateMustResolveToSignalObject=off  FilterRTWStateStorageClass=Auto  ParallelPVariant=InternalParameters  IdealPVariant=Disabled  IVariant=InternalParameters  DVariant=InternalParameters  IntegratorVariant=Continuous  SatVariant=Disabled  AWVariant=Passthrough  PCopyVariant=Disabled  TRVariant=Disabled  FdbkBlocksVariant=Forward  IdealPFdbkVariant=Disabled  SatFdbkVariant=Disabled  DerivativeFilterVariant=ContFilter  NVariant=InternalParameters  NCopyVariant=Disabled  FilterICVariant=InternalICsFilter  IntegratorICVariant=InternalICs  ExternalResetVariant=Disabled  TRSumVariant=Passthrough  SumFdbkVariant=Disabled  SumVariant=Sum_PID  TsampFilterVariant=InternalTs  TsampNgainVariant=Passthrough  TsampIntegralVariant=Disabled_SignalSpec  ExternalSaturationOutDataTypeStr=Inherit: Same as second input
  Sum1 : Sum  Inputs=|+-
  Sum19 : Sum  Inputs=|+-
  Sum2 : Sum  Inputs=|+-
  M1 : Outport
  M2 : Outport  Port=2
  M3 : Outport  Port=3
  wires:
  phidot/1 -> Sum19/2
  Sum19/1 -> PID Controller13/1
  Sum1/1 -> PID Controller12/1
  PID Controller12/1 -> M2/1
  psidot/1 -> Sum2/2
  Sum2/1 -> PID Controller14/1
  thetadot/1 -> Sum1/2
  PID Controller13/1 -> M1/1
  ref_phidot/1 -> Sum19/1
  ref_thetadot/1 -> Sum1/1
  ref_psidot/1 -> Sum2/1
  PID Controller14/1 -> M3/1

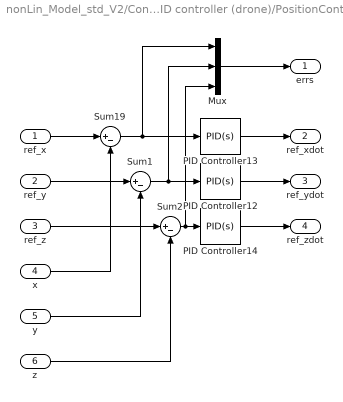
== system nonLin_Model_std_V2/Controllers/PID controller (drone)/PositionController ==
  ref_x : Inport
  ref_y : Inport  Port=2
  ref_z : Inport  Port=3
  x : Inport  Port=4
  y : Inport  Port=5
  z : Inport  Port=6
  Mux : Mux  Inputs=3
  PID Controller12 : slpidlib/PID Controller  Controller=PID  Form=Parallel  TimeDomain=Continuous-time  UseExternalTs=off  SampleTime=-1  IntegratorMethod=Forward Euler  FilterMethod=Forward Euler  ControllerParametersSource=internal  P=C.pos.y.Kp  I=C.pos.y.Ki  UseKiTs=off  D=C.pos.y.Kd  N=100  UseFilter=on  TunerSelectOption=Transfer Function Based (PID Tuner App)  InitialConditionSource=internal  InitialConditionForIntegrator=0  InitialConditionForFilter=0  DifferentiatorICPrevScaledInput=0  ExternalReset=none  TrackingMode=off  Kt=1  LimitOutput=off  SatLimitsSource=internal  UpperSaturationLimit=inf  LowerSaturationLimit=-inf  LinearizeAsGain=on  AntiWindupMode=none  Kb=1  LimitIntegrator=off  UpperIntegratorSaturationLimit=inf  LowerIntegratorSaturationLimit=-inf  POutMin=[]  POutMax=[]  IOutMin=[]  IOutMax=[]  DOutMin=[]  DOutMax=[]  NOutMin=[]  NOutMax=[]  SumOutMin=[]  SumOutMax=[]  SaturationOutMin=[]  SaturationOutMax=[]  PParamMin=[]  PParamMax=[]  IParamMin=[]  IParamMax=[]  DParamMin=[]  DParamMax=[]  NParamMin=[]  NParamMax=[]  KbParamMin=[]  KbParamMax=[]  KtParamMin=[]  KtParamMax=[]  KbOutMin=[]  KbOutMax=[]  KtOutMin=[]  KtOutMax=[]  IntegratorOutMin=[]  IntegratorOutMax=[]  FilterOutMin=[]  FilterOutMax=[]  SumI1OutMin=[]  SumI1OutMax=[]  SumI2OutMin=[]  SumI2OutMax=[]  SumI3OutMin=[]  SumI3OutMax=[]  SumI4OutMin=[]  SumI4OutMax=[]  SumDOutMin=[]  SumDOutMax=[]  DifferentiatorOutMin=[]  DifferentiatorOutMax=[]  FilterDiffOutCoefMin=[]  FilterDiffOutCoefMax=[]  ReciprocalOutMin=[]  ReciprocalOutMax=[]  SumDenOutMin=[]  SumDenOutMax=[]  SumNumOutMin=[]  SumNumOutMax=[]  DivideOutMin=[]  DivideOutMax=[]  UdiffTsProdOutMin=[]  UdiffTsProdOutMax=[]  NTsProdOutMin=[]  NTsProdOutMax=[]  UintegralTsProdOutMin=[]  UintegralTsProdOutMax=[]  UngainTsProdOutMin=[]  UngainTsProdOutMax=[]  ClampingZeroOutDataTypeStr=Inherit: Inherit via back propagation  ClampingZeroOutMin=[]  ClampingZeroOutMax=[]  FilterDenConstantOutDataTypeStr=Inherit: Inherit via back propagation  FilterDenConstantOutMin=[]  FilterDenConstantOutMax=[]  PCopyOutDataTypeStr=Inherit: Inherit via back propagation  PCopyOutMin=[]  PCopyOutMax=[]  NCopyOutDataTypeStr=Inherit: Inherit via back propagation  NCopyOutMin=[]  NCopyOutMax=[]  IntegratorContinuousStateAttributes=''  IntegratorStateMustResolveToSignalObject=off  IntegratorRTWStateStorageClass=Auto  FilterContinuousStateAttributes=''  FilterStateMustResolveToSignalObject=off  FilterRTWStateStorageClass=Auto  ParallelPVariant=InternalParameters  IdealPVariant=Disabled  IVariant=InternalParameters  DVariant=InternalParameters  IntegratorVariant=Continuous  SatVariant=Disabled  AWVariant=Passthrough  PCopyVariant=Disabled  TRVariant=Disabled  FdbkBlocksVariant=Forward  IdealPFdbkVariant=Disabled  SatFdbkVariant=Disabled  DerivativeFilterVariant=ContFilter  NVariant=InternalParameters  NCopyVariant=Disabled  FilterICVariant=InternalICsFilter  IntegratorICVariant=InternalICs  ExternalResetVariant=Disabled  TRSumVariant=Passthrough  SumFdbkVariant=Disabled  SumVariant=Sum_PID  TsampFilterVariant=InternalTs  TsampNgainVariant=Passthrough  TsampIntegralVariant=Disabled_SignalSpec  ExternalSaturationOutDataTypeStr=Inherit: Same as second input
  PID Controller13 : slpidlib/PID Controller  Controller=PID  Form=Parallel  TimeDomain=Continuous-time  UseExternalTs=off  SampleTime=-1  IntegratorMethod=Forward Euler  FilterMethod=Forward Euler  ControllerParametersSource=internal  P=C.pos.x.Kp  I=C.pos.x.Ki  UseKiTs=off  D=C.pos.x.Kd  N=100  UseFilter=on  TunerSelectOption=Transfer Function Based (PID Tuner App)  InitialConditionSource=internal  InitialConditionForIntegrator=0  InitialConditionForFilter=0  DifferentiatorICPrevScaledInput=0  ExternalReset=none  TrackingMode=off  Kt=1  LimitOutput=off  SatLimitsSource=internal  UpperSaturationLimit=inf  LowerSaturationLimit=-inf  LinearizeAsGain=on  AntiWindupMode=none  Kb=1  LimitIntegrator=off  UpperIntegratorSaturationLimit=inf  LowerIntegratorSaturationLimit=-inf  POutMin=[]  POutMax=[]  IOutMin=[]  IOutMax=[]  DOutMin=[]  DOutMax=[]  NOutMin=[]  NOutMax=[]  SumOutMin=[]  SumOutMax=[]  SaturationOutMin=[]  SaturationOutMax=[]  PParamMin=[]  PParamMax=[]  IParamMin=[]  IParamMax=[]  DParamMin=[]  DParamMax=[]  NParamMin=[]  NParamMax=[]  KbParamMin=[]  KbParamMax=[]  KtParamMin=[]  KtParamMax=[]  KbOutMin=[]  KbOutMax=[]  KtOutMin=[]  KtOutMax=[]  IntegratorOutMin=[]  IntegratorOutMax=[]  FilterOutMin=[]  FilterOutMax=[]  SumI1OutMin=[]  SumI1OutMax=[]  SumI2OutMin=[]  SumI2OutMax=[]  SumI3OutMin=[]  SumI3OutMax=[]  SumI4OutMin=[]  SumI4OutMax=[]  SumDOutMin=[]  SumDOutMax=[]  DifferentiatorOutMin=[]  DifferentiatorOutMax=[]  FilterDiffOutCoefMin=[]  FilterDiffOutCoefMax=[]  ReciprocalOutMin=[]  ReciprocalOutMax=[]  SumDenOutMin=[]  SumDenOutMax=[]  SumNumOutMin=[]  SumNumOutMax=[]  DivideOutMin=[]  DivideOutMax=[]  UdiffTsProdOutMin=[]  UdiffTsProdOutMax=[]  NTsProdOutMin=[]  NTsProdOutMax=[]  UintegralTsProdOutMin=[]  UintegralTsProdOutMax=[]  UngainTsProdOutMin=[]  UngainTsProdOutMax=[]  ClampingZeroOutDataTypeStr=Inherit: Inherit via back propagation  ClampingZeroOutMin=[]  ClampingZeroOutMax=[]  FilterDenConstantOutDataTypeStr=Inherit: Inherit via back propagation  FilterDenConstantOutMin=[]  FilterDenConstantOutMax=[]  PCopyOutDataTypeStr=Inherit: Inherit via back propagation  PCopyOutMin=[]  PCopyOutMax=[]  NCopyOutDataTypeStr=Inherit: Inherit via back propagation  NCopyOutMin=[]  NCopyOutMax=[]  IntegratorContinuousStateAttributes=''  IntegratorStateMustResolveToSignalObject=off  IntegratorRTWStateStorageClass=Auto  FilterContinuousStateAttributes=''  FilterStateMustResolveToSignalObject=off  FilterRTWStateStorageClass=Auto  ParallelPVariant=InternalParameters  IdealPVariant=Disabled  IVariant=InternalParameters  DVariant=InternalParameters  IntegratorVariant=Continuous  SatVariant=Disabled  AWVariant=Passthrough  PCopyVariant=Disabled  TRVariant=Disabled  FdbkBlocksVariant=Forward  IdealPFdbkVariant=Disabled  SatFdbkVariant=Disabled  DerivativeFilterVariant=ContFilter  NVariant=InternalParameters  NCopyVariant=Disabled  FilterICVariant=InternalICsFilter  IntegratorICVariant=InternalICs  ExternalResetVariant=Disabled  TRSumVariant=Passthrough  SumFdbkVariant=Disabled  SumVariant=Sum_PID  TsampFilterVariant=InternalTs  TsampNgainVariant=Passthrough  TsampIntegralVariant=Disabled_SignalSpec  ExternalSaturationOutDataTypeStr=Inherit: Same as second input
  PID Controller14 : slpidlib/PID Controller  Controller=PID  Form=Parallel  TimeDomain=Continuous-time  UseExternalTs=off  SampleTime=-1  IntegratorMethod=Forward Euler  FilterMethod=Forward Euler  ControllerParametersSource=internal  P=C.pos.z.Kp  I=C.pos.z.Ki  UseKiTs=off  D=C.pos.z.Kd  N=100  UseFilter=on  TunerSelectOption=Transfer Function Based (PID Tuner App)  InitialConditionSource=internal  InitialConditionForIntegrator=0  InitialConditionForFilter=0  DifferentiatorICPrevScaledInput=0  ExternalReset=none  TrackingMode=off  Kt=1  LimitOutput=off  SatLimitsSource=internal  UpperSaturationLimit=inf  LowerSaturationLimit=-inf  LinearizeAsGain=on  AntiWindupMode=none  Kb=1  LimitIntegrator=off  UpperIntegratorSaturationLimit=inf  LowerIntegratorSaturationLimit=-inf  POutMin=[]  POutMax=[]  IOutMin=[]  IOutMax=[]  DOutMin=[]  DOutMax=[]  NOutMin=[]  NOutMax=[]  SumOutMin=[]  SumOutMax=[]  SaturationOutMin=[]  SaturationOutMax=[]  PParamMin=[]  PParamMax=[]  IParamMin=[]  IParamMax=[]  DParamMin=[]  DParamMax=[]  NParamMin=[]  NParamMax=[]  KbParamMin=[]  KbParamMax=[]  KtParamMin=[]  KtParamMax=[]  KbOutMin=[]  KbOutMax=[]  KtOutMin=[]  KtOutMax=[]  IntegratorOutMin=[]  IntegratorOutMax=[]  FilterOutMin=[]  FilterOutMax=[]  SumI1OutMin=[]  SumI1OutMax=[]  SumI2OutMin=[]  SumI2OutMax=[]  SumI3OutMin=[]  SumI3OutMax=[]  SumI4OutMin=[]  SumI4OutMax=[]  SumDOutMin=[]  SumDOutMax=[]  DifferentiatorOutMin=[]  DifferentiatorOutMax=[]  FilterDiffOutCoefMin=[]  FilterDiffOutCoefMax=[]  ReciprocalOutMin=[]  ReciprocalOutMax=[]  SumDenOutMin=[]  SumDenOutMax=[]  SumNumOutMin=[]  SumNumOutMax=[]  DivideOutMin=[]  DivideOutMax=[]  UdiffTsProdOutMin=[]  UdiffTsProdOutMax=[]  NTsProdOutMin=[]  NTsProdOutMax=[]  UintegralTsProdOutMin=[]  UintegralTsProdOutMax=[]  UngainTsProdOutMin=[]  UngainTsProdOutMax=[]  ClampingZeroOutDataTypeStr=Inherit: Inherit via back propagation  ClampingZeroOutMin=[]  ClampingZeroOutMax=[]  FilterDenConstantOutDataTypeStr=Inherit: Inherit via back propagation  FilterDenConstantOutMin=[]  FilterDenConstantOutMax=[]  PCopyOutDataTypeStr=Inherit: Inherit via back propagation  PCopyOutMin=[]  PCopyOutMax=[]  NCopyOutDataTypeStr=Inherit: Inherit via back propagation  NCopyOutMin=[]  NCopyOutMax=[]  IntegratorContinuousStateAttributes=''  IntegratorStateMustResolveToSignalObject=off  IntegratorRTWStateStorageClass=Auto  FilterContinuousStateAttributes=''  FilterStateMustResolveToSignalObject=off  FilterRTWStateStorageClass=Auto  ParallelPVariant=InternalParameters  IdealPVariant=Disabled  IVariant=InternalParameters  DVariant=InternalParameters  IntegratorVariant=Continuous  SatVariant=Disabled  AWVariant=Passthrough  PCopyVariant=Disabled  TRVariant=Disabled  FdbkBlocksVariant=Forward  IdealPFdbkVariant=Disabled  SatFdbkVariant=Disabled  DerivativeFilterVariant=ContFilter  NVariant=InternalParameters  NCopyVariant=Disabled  FilterICVariant=InternalICsFilter  IntegratorICVariant=InternalICs  ExternalResetVariant=Disabled  TRSumVariant=Passthrough  SumFdbkVariant=Disabled  SumVariant=Sum_PID  TsampFilterVariant=InternalTs  TsampNgainVariant=Passthrough  TsampIntegralVariant=Disabled_SignalSpec  ExternalSaturationOutDataTypeStr=Inherit: Same as second input
  Sum1 : Sum  Inputs=|+-
  Sum19 : Sum  Inputs=|+-
  Sum2 : Sum  Inputs=|+-
  errs : Outport
  ref_xdot : Outport  Port=2
  ref_ydot : Outport  Port=3
  ref_zdot : Outport  Port=4
  wires:
  x/1 -> Sum19/2
  Sum19/1 -> Mux/1, PID Controller13/1
  Sum1/1 -> Mux/2, PID Controller12/1
  PID Controller12/1 -> ref_ydot/1
  z/1 -> Sum2/2
  Sum2/1 -> Mux/3, PID Controller14/1
  y/1 -> Sum1/2
  PID Controller13/1 -> ref_xdot/1
  ref_x/1 -> Sum19/1
  ref_y/1 -> Sum1/1
  ref_z/1 -> Sum2/1
  PID Controller14/1 -> ref_zdot/1
  Mux/1 -> errs/1
